simulink library "lib_Clutchless_HSC_ETE"  (R2017b)
settings: Solver=VariableStepAuto  StartTime=0.0  StopTime=10.0  RelTol=1e-3
undefined symbols (not defined in the file): cal, eng, Engine, ENGTRQ_MSMCH_Degraded_CP, ENGTRQ_MSMCH_ErrCritical_CP, ENGTRQ_MSMCH_LimpHome_CP, gb, mot, tloop
libraries: simulink x78, EC2_libraries x4, powerlib_meascontrol x2, lib_SystemDiag x1, dspsigops x1
(part 1 of 5)
settings Model: Creator=Di Russo  LastModifiedBy=Lyu19

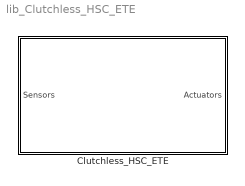
== system lib_Clutchless_HSC_ETE ==
  Clutchless_HSC_ETE : Subsystem
      mask Display: image('Images/HCU.jpg')

== system lib_Clutchless_HSC_ETE/Clutchless_HSC_ETE ==
  Sensors : Inport
  HSC : Subsystem
  Actuators : Outport
  wires:
  HSC/1(Actuators) -> Actuators/1
  Sensors/1 -> HSC/1(Sensors)

== system lib_Clutchless_HSC_ETE/Clutchless_HSC_ETE/HSC ==
  Sensors : Inport
  Camaro Fault Detection : Subsystem
  Driver_Requests : Subsystem  RequirementInfo="{'other' 'HCU_Requirements.xlsx' '@Simulink_requirement_item_5' 'true' 'Determines the  driver''s intention i.e. status of the vehicle start, HCU on/off status and the Driver Intend Axle Torque from the sensor inputs.' '' } %GIDa_ee5d0f02_0a71_4952_8ea3_2a40744828e3"
  Powertrain Manager : Subsystem
  Actuators : Outport
  wires:
  Driver_Requests/1(DriverRequests) -> Powertrain Manager/2(Driver Request)
  Camaro Fault Detection/1(Diagnostic) -> Driver_Requests/2("Diagnostic "), Powertrain Manager/3(Fault Detection)
  Powertrain Manager/1(Out1) -> Actuators/1
  Sensors/1 -> Driver_Requests/1(Sensors), Powertrain Manager/1(Sensors), Camaro Fault Detection/1(Sensors)
  Powertrain Manager/2(Controls) -> Driver_Requests/3("Controls ")

== system lib_Clutchless_HSC_ETE/Clutchless_HSC_ETE/HSC/Camaro Fault Detection ==
  Sensors : Inport
  Component Diagnostic : Subsystem
  Input Conversions : Subsystem
  Signal Diagnostic : Subsystem
  SystemDiag : lib_SystemDiag/SystemDiag
  Diagnostic : Outport
  wires:
  SystemDiag/1 -> Diagnostic/1
  Sensors/1 -> Input Conversions/1(RawSig)
  Input Conversions/1(VehSig) -> Signal Diagnostic/1(VehSig)
  Component Diagnostic/1(CompDiag) -> SystemDiag/1
  Signal Diagnostic/1(SignalDiag) -> Component Diagnostic/1(SignalDiag)

== system lib_Clutchless_HSC_ETE/Clutchless_HSC_ETE/HSC/Driver_Requests ==
  note: Driver management
  Sensors : Inport
  "Diagnostic " : Inport  Port=2
  "Controls " : Inport  Port=3
  APP_BPP to DrvIntndAxlTrq2 : Subsystem
  DriverRequests : Outport
  wires:
  Sensors/1 -> APP_BPP to DrvIntndAxlTrq2/1(Sensors)
  APP_BPP to DrvIntndAxlTrq2/1(IntndAxlTrq) -> DriverRequests/1
  "Diagnostic "/1 -> APP_BPP to DrvIntndAxlTrq2/2(Diag)
  "Controls "/1 -> APP_BPP to DrvIntndAxlTrq2/3(Controls)

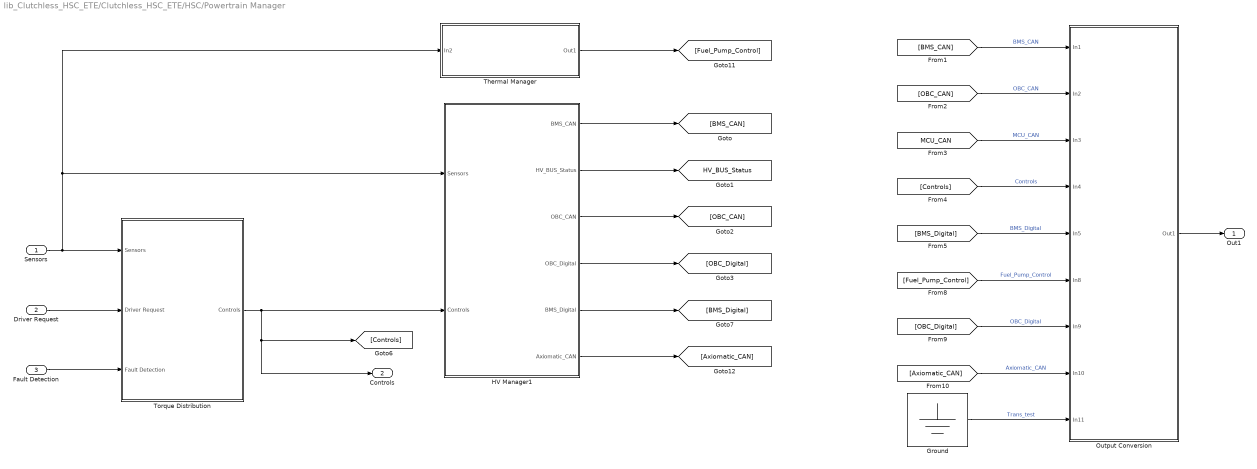
== system lib_Clutchless_HSC_ETE/Clutchless_HSC_ETE/HSC/Powertrain Manager ==
  Sensors : Inport
  Driver Request : Inport  Port=2
  Fault Detection : Inport  Port=3
  Ground : Ground
  HV Manager1 : Subsystem  AncestorBlock=lib_HVManager_PostIMG_2017a/HV Manager
  Output Conversion : Subsystem
  Thermal Manager : Subsystem  AncestorBlock=lib_ThermalManager/Thermal Manager
  Torque Distribution : Subsystem  AncestorBlock=lib_TorqueDistribution_2017a/Torque Distribution
  Out1 : Outport
  Controls : Outport  Port=2
  tag scope: HV_BUS_Status=global
  wires:
  Sensors/1 -> Torque Distribution/1(Sensors), HV Manager1/1(Sensors), Thermal Manager/1(In2)
  [Fuel_Pump_Control] -> Output Conversion/6(In8)  "Fuel_Pump_Control"
  [OBC_Digital] -> Output Conversion/7(In9)  "OBC_Digital"
  [Axiomatic_CAN] -> Output Conversion/8(In10)  "Axiomatic_CAN"
  HV Manager1/6(Axiomatic_CAN) -> [Axiomatic_CAN]
  Thermal Manager/1(Out1) -> [Fuel_Pump_Control]
  Fault Detection/1 -> Torque Distribution/3(Fault Detection)
  [BMS_Digital] -> Output Conversion/5(In5)  "BMS_Digital"
  HV Manager1/5(BMS_Digital) -> [BMS_Digital]
  Output Conversion/1(Out1) -> Out1/1
  [Controls] -> Output Conversion/4(In4)  "Controls"
  [MCU_CAN] -> Output Conversion/3(In3)  "MCU_CAN"
  [OBC_CAN] -> Output Conversion/2(In2)  "OBC_CAN"
  [BMS_CAN] -> Output Conversion/1(In1)  "BMS_CAN"
  Driver Request/1 -> Torque Distribution/2(Driver Request)
  HV Manager1/3(OBC_CAN) -> [OBC_CAN]
  HV Manager1/4(OBC_Digital) -> [OBC_Digital]
  HV Manager1/2(HV_BUS_Status) -> [HV_BUS_Status]
  HV Manager1/1(BMS_CAN) -> [BMS_CAN]
  Ground/1 -> Output Conversion/9(In11)  "Trans_test"
  Torque Distribution/1(Controls) -> HV Manager1/2(Controls), Controls/1, [Controls]

== system lib_Clutchless_HSC_ETE/Clutchless_HSC_ETE/HSC/Camaro Fault Detection/Component Diagnostic ==
  note: Component Diagnostics
  note: Component Status Setting Rule
      | xxx_CompStatus could be 0, 1, 2 or 3
      | 0: component needs to be offline
      | 1: component needs torque plant to deliver creep torque
      | 2: component needs torque plant to limit maximum torque delivery
      | 3: component needs torque plant to operate normally
  SignalDiag : Inport
  Bus Creator : BusCreator  Inputs=6
  Driver Input Diagnostic : Subsystem
  ESS Component Diagnostic : Subsystem
  Engine Component Diagnostic : Subsystem
  Override Driver Status : Subsystem
  Override ESS Status : Subsystem
  Override Engine Status : Subsystem
  Override TCM Status : Subsystem
  Transmission Component Diagnostic : Subsystem
  CompDiag : Outport
  wires:
  Engine Component Diagnostic/2(Out2) -> Bus Creator/4  "EngTrqMismchType"
  Override Driver Status/1(Out1) -> Bus Creator/1  "Driver_Input_Status"
  Override TCM Status/1(Out1) -> Bus Creator/5  "TCM_Status"
  Override Engine Status/1(Out1) -> Bus Creator/3  "ECM_Status"
  Override ESS Status/1(Out1) -> Bus Creator/2  "BMS_Status"
  Transmission Component Diagnostic/1(Out1) -> Override TCM Status/1(In1)  "TCM_CompDiag"
  Engine Component Diagnostic/1(Out1) -> Override Engine Status/1(In1)  "ECM_CompDiag"
  ESS Component Diagnostic/1(Out1) -> Override ESS Status/1(In1)  "ESS_CompDiag"
  Driver Input Diagnostic/1(Out1) -> Override Driver Status/1(In1)  "Diver_CompDiag"
  Bus Creator/1 -> CompDiag/1
  SignalDiag/1 -> Driver Input Diagnostic/1(In1), ESS Component Diagnostic/1(In1), Bus Creator/6, Transmission Component Diagnostic/1(In1), Engine Component Diagnostic/1(In1)  "RawSig"

== system lib_Clutchless_HSC_ETE/Clutchless_HSC_ETE/HSC/Camaro Fault Detection/Input Conversions ==
  note: These subsystems convert variable types to match those used in the
      | supervisor. In addition, override switches installed on each signal can
      | be used to manually override and signal for testing purposes
  note: Input Conversions and Override Switches
  RawSig : Inport
  BMS_Conversions : Subsystem
  Bus Creator : BusCreator  Inputs=5
  DriverInput_Conversions : Subsystem
  ECM_Conversions : Subsystem
  TCM_Conversions : Subsystem
  VehSig : Outport
  wires:
  TCM_Conversions/1(Out1) -> Bus Creator/4
  ECM_Conversions/1(Out1) -> Bus Creator/3
  RawSig/1 -> BMS_Conversions/1(In1), ECM_Conversions/1(In1), TCM_Conversions/1(In1), Bus Creator/5, DriverInput_Conversions/1(In1)  "RawSig"
  BMS_Conversions/1(Out1) -> Bus Creator/2
  Bus Creator/1 -> VehSig/1  "InputConvAndOvrd"
  DriverInput_Conversions/1(Out1) -> Bus Creator/1

== system lib_Clutchless_HSC_ETE/Clutchless_HSC_ETE/HSC/Camaro Fault Detection/Signal Diagnostic ==
  note: Signal Diagnostics
  note: These subsystems evaluate each signal for proper value range and other checks
  VehSig : Inport
  Bus Creator : BusCreator  Inputs=5
  Driver Signal Diagnostic : Subsystem
  ESS Signal Diagnostic : Subsystem
  Engine Signal Diagnostic : Subsystem
  Subsystem1 : Subsystem
      mask Display: fprintf('Signal Naming Rule')
  Transmission Signal Diagnostic : Subsystem
  SignalDiag : Outport
  wires:
  Bus Creator/1 -> SignalDiag/1  "SignalDiag"
  Transmission Signal Diagnostic/1(Out2) -> Bus Creator/4  "Transmission_SigDiag"
  Engine Signal Diagnostic/1(Engine_SigDiag) -> Bus Creator/3  "Engine_SigDiag"
  ESS Signal Diagnostic/1(ESS_SigDiag) -> Bus Creator/2  "ESS_SigDiag"
  Driver Signal Diagnostic/1(Driver_SigDiag) -> Bus Creator/1  "Driver_SigDiag"
  VehSig/1 -> Transmission Signal Diagnostic/1(Sensors1), Bus Creator/5, Engine Signal Diagnostic/1(Sensors1), Driver Signal Diagnostic/1(Sensors1), ESS Signal Diagnostic/1(Sensors1)

== system lib_Clutchless_HSC_ETE/Clutchless_HSC_ETE/HSC/Driver_Requests/APP_BPP to DrvIntndAxlTrq2 ==
  note: Note:Driver requested Axle Torque Calculation
  note: $Author: fy6949 $
      | $Rev: 577 $
      | $Date: 2017-1-19 08:53:15 -0500  $
  Sensors : Inport
  Diag : Inport  Port=2
  Controls : Inport  Port=3
  Bus Selector : BusSelector  OutputSignals=from_Analog.Driver_APP1,from_CAN.fromVEH_CAN.from_BCM.BrkPdlPos,from_CAN.fromEBCAN.from_ECM.VehSpdAvgDrvn,from_CAN.fromVEH_CAN.from_TCM.TrnGrRat,from_CAN.fromHV_CAN.from_MCU.INV_VCU_01.INV_Speed
  Bus Selector1 : BusSelector  OutputSignals=CompSig.RawSig.Driver_SigDiag.Drv_APP_Agree
  Bus Selector2 : BusSelector  OutputSignals=mode
  Post Driver Intnded Axle Torque : Subsystem
  Terminator : Terminator
  Terminator1 : Terminator
  IntndAxlTrq : Outport
  wires:
  Sensors/1 -> Bus Selector/1
  Controls/1 -> Bus Selector2/1
  Post Driver Intnded Axle Torque/1(IntndAxlTrq) -> IntndAxlTrq/1
  Bus Selector/2 -> Post Driver Intnded Axle Torque/2(BPP)  "<BrkPdlPos>"
  Bus Selector/3 -> Post Driver Intnded Axle Torque/3(VehicleSpeed)  "<VehSpdAvgDrvn>"
  Bus Selector/5 -> Post Driver Intnded Axle Torque/6(Motor_Speed)  "<INV_Speed>"
  Bus Selector/4 -> Post Driver Intnded Axle Torque/4(TransGearRatio)  "<TrnGrRat>"
  Bus Selector/1 -> Post Driver Intnded Axle Torque/1(APP)  "<Driver_APP1>"
  Post Driver Intnded Axle Torque/2(BrkIntndAxlTrq) -> Terminator/1
  Diag/1 -> Bus Selector1/1
  Bus Selector1/1 -> Terminator1/1  "<Drv_APP_Agree>"
  Bus Selector2/1 -> Post Driver Intnded Axle Torque/5(Mode)  "<mode>"

== system lib_Clutchless_HSC_ETE/Clutchless_HSC_ETE/HSC/Powertrain Manager/HV Manager1 ==
  Sensors : Inport
  Controls : Inport  Port=2
  Axiomatic_Output_Manager : Subsystem
  BMS_Manager : Subsystem
  Bus Creator1 : BusCreator  Inputs=4
  DCDC Manager : Subsystem
  Inverter Manager : Subsystem
  OBC_Manager : Subsystem
  BMS_CAN : Outport
  HV_BUS_Status : Outport  Port=2
  OBC_CAN : Outport  Port=3
  OBC_Digital : Outport  Port=4
  BMS_Digital : Outport  Port=5
  Axiomatic_CAN : Outport  Port=6
  tag scope: MCU_CAN=global
  wires:
  Bus Creator1/1 -> [MCU_CAN]
  Inverter Manager/2(MCU_CAN) -> Bus Creator1/2  "MCU_CAN"
  Inverter Manager/1(MCU_Status) -> [MCU_Status], Bus Creator1/1  "MCU_Status"
  Sensors/1 -> BMS_Manager/1(Sensors), DCDC Manager/1(BMSInput), Axiomatic_Output_Manager/1(Sensors), OBC_Manager/2(Sensors), Inverter Manager/2(Sensors)
  [HV_BUS_Status] -> Inverter Manager/1(HV_Bus_Status)  "HV_BUS_Status"
  [HV_BUS_Status] -> Axiomatic_Output_Manager/2(HV_Bus_Status)
  BMS_Manager/2(HV_BUS_Status) -> [HV_BUS_Status], HV_BUS_Status/1  "HV_BUS_Status"
  [HV_BUS_Status] -> OBC_Manager/1(HV_Status)
  OBC_Manager/1(OBC CAN) -> OBC_CAN/1
  OBC_Manager/2(OBC_Digital) -> OBC_Digital/1
  Controls/1 -> BMS_Manager/2(Controls), DCDC Manager/2(In1), DCDC Manager/3(In2), Inverter Manager/3(Control)
  BMS_Manager/1(BMS CAN) -> BMS_CAN/1
  BMS_Manager/3(BMS Digital) -> BMS_Digital/1
  Axiomatic_Output_Manager/1(Axiomatic_CAN) -> Axiomatic_CAN/1
  Inverter Manager/3(MCU_Relay) -> Bus Creator1/3  "MCU_Relay"
  DCDC Manager/1(Out1) -> Bus Creator1/4
  [MCU_Status] -> BMS_Manager/3(In1)

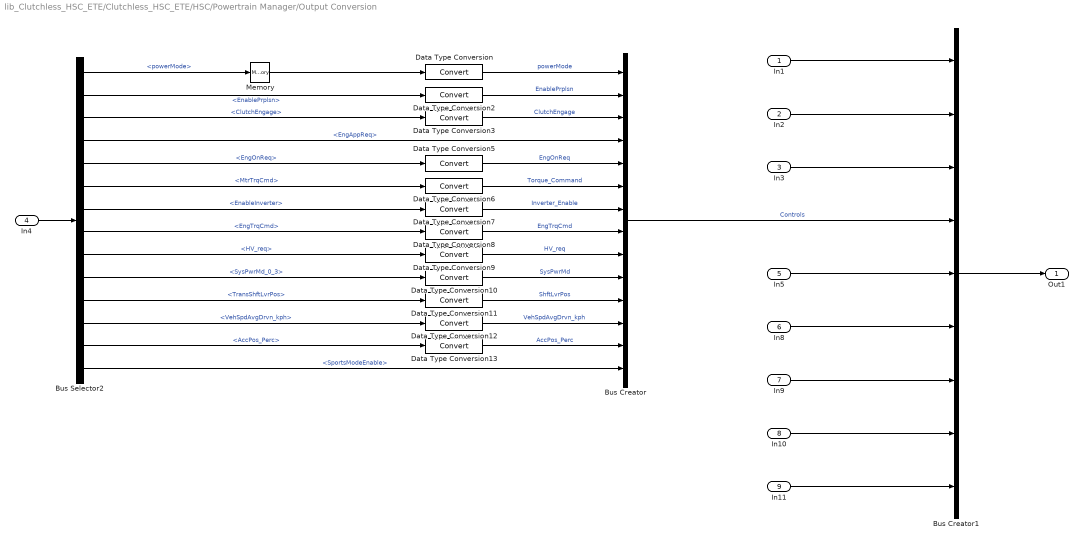
== system lib_Clutchless_HSC_ETE/Clutchless_HSC_ETE/HSC/Powertrain Manager/Output Conversion ==
  In1 : Inport
  In2 : Inport  Port=2
  In3 : Inport  Port=3
  In4 : Inport  Port=4
  In5 : Inport  Port=5
  In8 : Inport  Port=6
  In9 : Inport  Port=7
  In10 : Inport  Port=8
  In11 : Inport  Port=9
  Bus Creator : BusCreator  Inputs=14
  Bus Creator1 : BusCreator  Inputs=9
  Bus Selector2 : BusSelector  OutputSignals=powerMode,EnablePrplsn,ClutchEngage,EngAppReq,EngOnReq,MtrTrqCmd,EnableInverter,EngTrqCmd,HV_req,SysPwrMd_0_3,TransShftLvrPos,VehSpdAvgDrvn_kph,AccPos_Perc,SportsModeEnable
  Data Type Conversion{,2..3,5..13} (12 alike) : DataTypeConversion
  Memory : Memory
  Out1 : Outport
  wires:
  In10/1 -> Bus Creator1/8
  In9/1 -> Bus Creator1/7
  In8/1 -> Bus Creator1/6
  Memory/1 -> Data Type Conversion/1
  Data Type Conversion13/1 -> Bus Creator/13  "AccPos_Perc"
  Bus Selector2/13 -> Data Type Conversion13/1  "<AccPos_Perc>"
  Data Type Conversion12/1 -> Bus Creator/12  "VehSpdAvgDrvn_kph"
  Bus Selector2/12 -> Data Type Conversion12/1  "<VehSpdAvgDrvn_kph>"
  Data Type Conversion11/1 -> Bus Creator/11  "ShftLvrPos"
  Bus Selector2/11 -> Data Type Conversion11/1  "<TransShftLvrPos>"
  In5/1 -> Bus Creator1/5
  Bus Creator/1 -> Bus Creator1/4  "Controls"
  In3/1 -> Bus Creator1/3
  In2/1 -> Bus Creator1/2
  In1/1 -> Bus Creator1/1
  Bus Creator1/1 -> Out1/1
  Data Type Conversion5/1 -> Bus Creator/5  "EngOnReq"
  Data Type Conversion/1 -> Bus Creator/1  "powerMode"
  Data Type Conversion10/1 -> Bus Creator/10  "SysPwrMd"
  Data Type Conversion9/1 -> Bus Creator/9  "HV_req"
  Data Type Conversion8/1 -> Bus Creator/8  "EngTrqCmd"
  Data Type Conversion7/1 -> Bus Creator/7  "Inverter_Enable"
  Data Type Conversion6/1 -> Bus Creator/6  "Torque_Command"
  Bus Selector2/4 -> Bus Creator/4  "<EngAppReq>"
  Data Type Conversion3/1 -> Bus Creator/3  "ClutchEngage"
  Data Type Conversion2/1 -> Bus Creator/2  "EnablePrplsn"
  Bus Selector2/10 -> Data Type Conversion10/1  "<SysPwrMd_0_3>"
  Bus Selector2/9 -> Data Type Conversion9/1  "<HV_req>"
  Bus Selector2/8 -> Data Type Conversion8/1  "<EngTrqCmd>"
  Bus Selector2/7 -> Data Type Conversion7/1  "<EnableInverter>"
  Bus Selector2/6 -> Data Type Conversion6/1  "<MtrTrqCmd>"
  Bus Selector2/5 -> Data Type Conversion5/1  "<EngOnReq>"
  Bus Selector2/3 -> Data Type Conversion3/1  "<ClutchEngage>"
  Bus Selector2/2 -> Data Type Conversion2/1  "<EnablePrplsn>"
  Bus Selector2/1 -> Memory/1  "<powerMode>"
  In4/1 -> Bus Selector2/1
  In11/1 -> Bus Creator1/9
  Bus Selector2/14 -> Bus Creator/14  "<SportsModeEnable>"

== system lib_Clutchless_HSC_ETE/Clutchless_HSC_ETE/HSC/Powertrain Manager/Thermal Manager ==
  In2 : Inport
  Bus Creator : BusCreator  Inputs=3
  Bus Creator1 : BusCreator  Inputs=4
  Bus Creator2 : BusCreator  Inputs=4
  Bus Creator3 : BusCreator  Inputs=3
  Bus Creator4 : BusCreator  Inputs=1
  Bus Selector : BusSelector  OutputSignals=from_CAN.fromEBCAN.from_ECM.EngCltTmp,from_CAN.fromHV_CAN.from_BMSHybrid.BMS_Temperatur,from_CAN.fromHV_CAN.from_MCU.INV_VCU_04.INV_InverterTemperature,from_CAN.fromHV_CAN.from_MCU.INV_VCU_04.INV_ElectricMachineTemperature,from_CAN.fromEBCAN.from_ECM.EngRunAtv,from_CAN.fromHV_CAN.from_BMSHybrid.BMS_HYB_02.BMS_IstModus,from_CAN.fromVEH_CAN.from_BCM.SysPwrMd,from_CAN.fromEBCAN.from_ECM.VehSpdAvgDrvn
  Bus Selector3 : BusSelector  OutputSignals=from_CAN.fromHV_CAN.from_BMSHybrid.BMS_HYB_02.BMS_Fehler_Pilot
  Compare To Constant1 : simulink/Logic and Bit Operations/Compare To Constant  relop=>  const=0  OutDataTypeStr=boolean
  Cooling Fan Manger : Subsystem
  Data Type Conversion : DataTypeConversion  OutDataTypeStr=double
  ESS Pump Manger : Subsystem
  MotInv Pump Manger : Subsystem
  Out1 : Outport
  wires:
  Bus Selector/8 -> Bus Creator/3  "<VehSpdAvgDrvn>"
  Bus Selector/7 -> Bus Creator3/3  "<SysPwrMd>"
  Bus Selector/6 -> Bus Creator3/2  "<BMS_IstModus>"
  Bus Selector/5 -> Bus Creator3/1  "<EngRunAtv>"
  Bus Selector/4 -> Bus Creator2/4  "<INV_ElectricMachineTemperature>"
  Bus Selector/3 -> Bus Creator2/3  "<INV_InverterTemperature>"
  Bus Selector/2 -> Bus Creator2/2  "<BMS_Temperatur>"
  Bus Selector/1 -> Bus Creator2/1  "<EngCltTmp>"
  Bus Creator1/1 -> Out1/1  "Thermal_Control"
  Cooling Fan Manger/1(Fan_control) -> Bus Creator1/1  "Fan_Control"
  Bus Creator/1 -> Cooling Fan Manger/1(Temp), ESS Pump Manger/1(ESS_temp), MotInv Pump Manger/1(MotInv_temp)
  ESS Pump Manger/1(ESS_Thermal_Control) -> Bus Creator1/2  "ESS_Pump_Control"
  MotInv Pump Manger/1(MotInvpump_control) -> Bus Creator1/3  "MotMCU_Pump_Control"
  Bus Creator2/1 -> Bus Creator/1  "Temp_Signals"
  Bus Creator3/1 -> Bus Creator/2  "Component_State"
  In2/1 -> Bus Selector3/1, Bus Selector/1
  Bus Selector3/1 -> Compare To Constant1/1  "<BMS_Fehler_Pilot>"
  Bus Creator4/1 -> Bus Creator1/4  "Pump_Commands"
  Data Type Conversion/1 -> Bus Creator4/1  "FuelPump_Disable"
  Compare To Constant1/1 -> Data Type Conversion/1

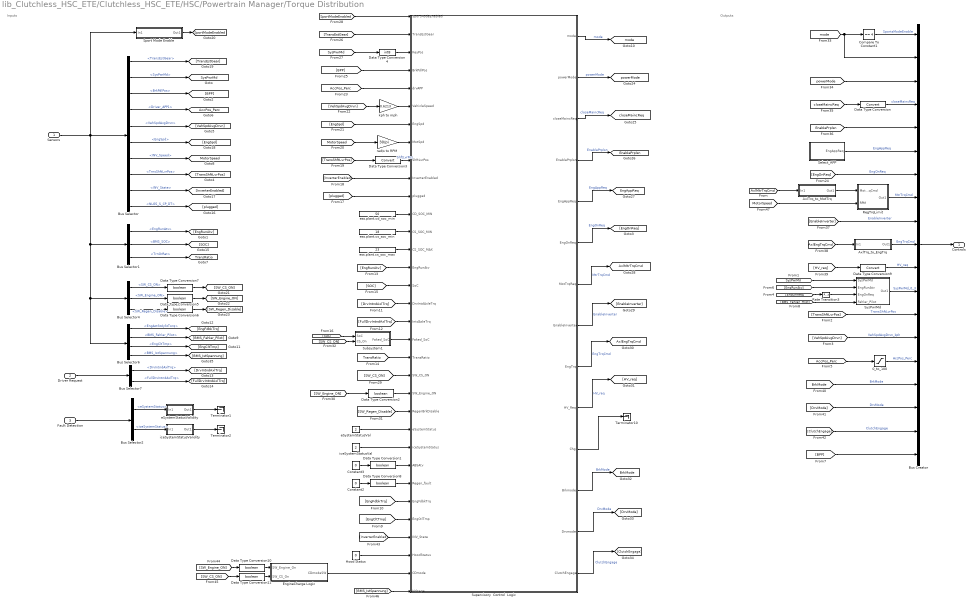
== system lib_Clutchless_HSC_ETE/Clutchless_HSC_ETE/HSC/Powertrain Manager/Torque Distribution ==
  note: Outputs
  note: Inputs
  Sensors : Inport
  Driver Request : Inport  Port=2
  Fault Detection : Inport  Port=3
  0_to_100 : Saturate  UpperLimit=100  LowerLimit=0
  AxlTrq_to_EngTrq : Subsystem
  AxlTrq_to_MotTrq : Subsystem
  Bus Creator : BusCreator  Inputs=19
  Bus Selector : BusSelector  OutputSignals=from_CAN.fromVEH_CAN.from_TCM.TransEstGear,from_CAN.fromVEH_CAN.from_BCM.SysPwrMd,from_CAN.fromVEH_CAN.from_BCM.BrkPdlPos,from_Analog.Driver_APP1,from_CAN.fromEBCAN.from_ECM.VehSpdAvgDrvn,from_CAN.fromEBCAN.from_ECM.EngSpd,from_CAN.fromHV_CAN.from_MCU.INV_VCU_01.INV_Speed,from_CAN.fromVEH_CAN.from_TCM.TrnsShftLvrPos,from_CAN.fromHV_CAN.from_MCU.INV_VCU_01.INV_State,from_CAN.fromHV_CAN.from_OBC.NLG5_ST.NLG5_S_CP_DT
  Bus Selector1 : BusSelector  OutputSignals=from_CAN.fromEBCAN.from_ECM.EngRunAtv,from_CAN.fromHV_CAN.from_BMSHybrid.BMS_SOC,from_CAN.fromVEH_CAN.from_TCM.TrnGrRat
  Bus Selector2 : BusSelector  OutputSignals=eSystemDiagOut.eSystemStatus,iceSystemDiagOut.iceSystemStatus
  Bus Selector4 : BusSelector  OutputSignals=from_Digital.SW_CS_ON,from_Digital.SW_Engine_ON,from_Digital.SW_Regen_Disable
  Bus Selector6 : BusSelector  OutputSignals=from_CAN.fromEBCAN.from_ECM.EngActStdyStTorq,from_CAN.fromHV_CAN.from_BMSHybrid.BMS_HYB_02.BMS_Fehler_Pilot,from_CAN.fromEBCAN.from_ECM.EngCltTmp,from_CAN.fromHV_CAN.from_BMSHybrid.BMS_HYB_02.BMS_IstSpannung
  Bus Selector7 : BusSelector  OutputSignals=DrvIntndAxlTrq,FullDrvIntndAxlTrq
  Compare To Constant1 : simulink/Logic and Bit Operations/Compare To Constant  relop===  const=4  OutDataTypeStr=boolean
  Constant2 : Constant  Value=0
  Constant3 : Constant  Value=0
  Data Type Conversion : DataTypeConversion
  Data Type Conversion{1..2,5..8,10..11} (8 alike) : DataTypeConversion  OutDataTypeStr=boolean
  Data Type Conversion3 : DataTypeConversion
  Data Type Conversion4 : DataTypeConversion  OutDataTypeStr=int8
  Data Type Conversion9 : DataTypeConversion
  EngineCharge Logic : Stateflow chart  TreatAsAtomicUnit=on
  Hood Status : Constant  Value=0
  Rate Transition3 : RateTransition
  RegTrqLimit : Subsystem
  Select_APP : Subsystem
  Sport Mode Enable : Subsystem
  Subsystem1 : Subsystem
  Supervisory  Control  Logic : Stateflow chart  TreatAsAtomicUnit=on
  SysPwrMd : Subsystem
  Terminator1 : Terminator
  Terminator10 : Terminator
  Terminator2 : Terminator
  eSystemStatusVal : Constant  Value=2
  eSystemStatusValidity : Subsystem
  ess.plant.cd_soc_min : Constant  Value=50
  ess.plant.cs_soc_max : Constant  Value=23
  ess.plant.cs_soc_min : Constant  Value=18
  iceSystemStatusVal : Constant  Value=2
  iceSystemStatusValidity : Subsystem
  kph to mph : Gain  Gain=0.6213
  rad/s to RPM : Gain  Gain=30/pi
  Controls : Outport
  tag scope: AccPos_Perc=global, AxlEngTrqCmd=global, AxlMtrTrqCmd=global, BrkMode=global, EnablePrplsn=global, EngAppReq=global, MotorSpeed=global, SportModeEnabled=global, SysPwrMd=global, TransRatio=global, closeMaincReq=global, mode=global, powerMode=global
  wires:
  [InverterEnabled] -> Supervisory  Control  Logic/30(INV_State)
  Data Type Conversion2/1 -> Supervisory  Control  Logic/22(SW_Engine_ON)
  [SW_Engine_ON] -> Data Type Conversion2/1
  ess.plant.cd_soc_min/1 -> Supervisory  Control  Logic/12(CD_SOC_MIN)
  ess.plant.cs_soc_min/1 -> Supervisory  Control  Logic/13(CS_SOC_MIN)
  ess.plant.cs_soc_max/1 -> Supervisory  Control  Logic/14(CS_SOC_MAX)
  Supervisory  Control  Logic/8(EnableInverter) -> [EnableInverter]  "EnableInverter"
  Supervisory  Control  Logic/4(EnablePrplsn) -> [EnablePrplsn]  "EnablePrplsn"
  Supervisory  Control  Logic/3(closeMaincReq) -> [closeMaincReq]  "closeMaincReq"
  Supervisory  Control  Logic/2(powerMode) -> [powerMode]  "powerMode"
  Supervisory  Control  Logic/1(mode) -> [mode]  "mode"
  Data Type Conversion3/1 -> Supervisory  Control  Logic/9(ShftLvrPos)  "ShftLvrPos"
  kph to mph/1 -> Supervisory  Control  Logic/6(VehicleSpeed)
  Constant2/1 -> Data Type Conversion8/1
  Supervisory  Control  Logic/11(Chg) -> Terminator10/1
  [DrvIntndAxlTrq] -> Supervisory  Control  Logic/17(DrvIntdAxleTrq)
  [FullDrvIntndAxlTrq] -> Supervisory  Control  Logic/18(IntdAxleTrq)
  Constant3/1 -> Data Type Conversion1/1
  Data Type Conversion1/1 -> Supervisory  Control  Logic/26(ABSAtv)
  Subsystem1/1(Faked_SoC) -> Supervisory  Control  Logic/19(Faked_SoC)
  Supervisory  Control  Logic/12(Brkmode) -> [BrkMode]  "BrkMode"
  Data Type Conversion8/1 -> Supervisory  Control  Logic/27(Regen_fault)
  iceSystemStatusVal/1 -> Supervisory  Control  Logic/25(iceSystemStatus)
  eSystemStatusVal/1 -> Supervisory  Control  Logic/24(eSystemStatus)
  Supervisory  Control  Logic/5(EngAppReq) -> [EngAppReq]  "EngAppReq"
  rad/s to RPM/1 -> Supervisory  Control  Logic/8(MotSpd)
  [EngCltTmp] -> Supervisory  Control  Logic/29(EngCtlTmp)
  [EngFdbkTrq] -> Supervisory  Control  Logic/28(EngFdbkTrq)
  [EngRunAtv] -> Supervisory  Control  Logic/15(EngRunAtv)
  [TransRatio] -> Supervisory  Control  Logic/20(TransRatio)
  [SOC] -> Supervisory  Control  Logic/16(SoC)
  [SOC] -> Subsystem1/1(SoC)
  [InverterEnabled] -> Supervisory  Control  Logic/10(InverterEnabled)
  [TransShftLvrPos] -> Data Type Conversion3/1
  [MotorSpeed] -> rad/s to RPM/1
  [EngSpd] -> Supervisory  Control  Logic/7(EngSpd)
  [VehSpdAvgDrvn] -> kph to mph/1
  [AccPos_Perc] -> Supervisory  Control  Logic/5(drvAPP)
  [BPP] -> Supervisory  Control  Logic/4(BrkPdlPos)
  [TransEstGear] -> Supervisory  Control  Logic/2(TransEstGear)
  [SysPwrMd] -> Data Type Conversion4/1
  Data Type Conversion4/1 -> Supervisory  Control  Logic/3(KeyPos)
  [SportModeEnabled] -> Supervisory  Control  Logic/1(SportModeEnabled)
  [SW_CS_ON] -> Supervisory  Control  Logic/21(SW_CS_ON)
  [SW_Regen_Disable] -> Supervisory  Control  Logic/23(RegenBrkDisable)
  [SW_CS_ON] -> Subsystem1/2(CS_On)
  Supervisory  Control  Logic/6(EngOnReq) -> [EngOnReq]  "EngOnReq"
  Supervisory  Control  Logic/7(MotTrqReq) -> [AxlMtrTrqCmd]  "MtrTrqCmd"
  Supervisory  Control  Logic/9(EngTrq) -> [AxlEngTrqCmd]  "EngTrqCmd"
  Supervisory  Control  Logic/10(HV_Req) -> [HV_req]  "HV_req"
  Supervisory  Control  Logic/13(Drvmode) -> [DrvMode]  "DrvMode"
  Supervisory  Control  Logic/14(ClutchEngage) -> [ClutchEngage]  "ClutchEngage"
  Bus Selector7/1 -> [DrvIntndAxlTrq]  "<DrvIntndAxlTrq>"
  Driver Request/1 -> Bus Selector7/1
  Data Type Conversion7/1 -> [SW_CS_ON]
  Bus Selector1/2 -> [SOC]  "<BMS_SOC>"
  Sport Mode Enable/1(Out1) -> [SportModeEnabled]
  Bus Selector7/2 -> [FullDrvIntndAxlTrq]  "<FullDrvIntndAxlTrq>"
  Bus Selector6/3 -> [EngCltTmp]  "<EngCltTmp>"
  Bus Selector6/2 -> [BMS_Fehler_Pilot]  "<BMS_Fehler_Pilot>"
  Bus Selector6/1 -> [EngFdbkTrq]  "<EngActStdyStTorq>"
  Data Type Conversion6/1 -> [SW_Regen_Disable]
  Data Type Conversion5/1 -> [SW_Engine_ON]
  Bus Selector/10 -> [plugged]  "<NLG5_S_CP_DT>"
  iceSystemStatusValidity/1(Out1) -> Terminator2/1
  eSystemStatusValidity/1(Out1) -> Terminator1/1
  Bus Selector4/2 -> Data Type Conversion5/1  "<SW_Engine_ON>"
  Bus Selector4/1 -> Data Type Conversion7/1  "<SW_CS_ON>"
  Bus Selector4/3 -> Data Type Conversion6/1  "<SW_Regen_Disable>"
  Bus Selector2/2 -> iceSystemStatusValidity/1(In1)  "<iceSystemStatus>"
  Bus Selector2/1 -> eSystemStatusValidity/1(In1)  "<eSystemStatus>"
  Fault Detection/1 -> Bus Selector2/1
  Bus Selector1/3 -> [TransRatio]  "<TrnGrRat>"
  Bus Selector/8 -> [TransShftLvrPos]  "<TrnsShftLvrPos>"
  Bus Selector1/1 -> [EngRunAtv]  "<EngRunAtv>"
  Bus Selector/9 -> [InverterEnabled]  "<INV_State>"
  Bus Selector/7 -> [MotorSpeed]  "<INV_Speed>"
  Bus Selector/6 -> [EngSpd]  "<EngSpd>"
  Bus Selector/5 -> [VehSpdAvgDrvn]  "<VehSpdAvgDrvn>"
  Bus Selector/4 -> [AccPos_Perc]  "<Driver_APP1>"
  Bus Selector/3 -> [BPP]  "<BrkPdlPos>"
  Bus Selector/2 -> [SysPwrMd]  "<SysPwrMd>"
  Bus Selector/1 -> [TransEstGear]  "<TransEstGear>"
  Sensors/1 -> Sport Mode Enable/1(In1), Bus Selector6/1, Bus Selector4/1, Bus Selector1/1, Bus Selector/1
  Bus Creator/1 -> Controls/1
  Rate Transition3/1 -> SysPwrMd/3(EngOnReq)
  [EngOnReq] -> Rate Transition3/1
  Data Type Conversion/1 -> Bus Creator/4  "closeMaincReq"
  [powerMode] -> Bus Creator/3
  0_to_100/1 -> Bus Creator/15  "AccPos_Perc"
  RegTrqLimit/1(Out1) -> Bus Creator/8  "MtrTrqCmd"
  [BrkMode] -> Bus Creator/16  "BrkMode"
  Select_APP/1(EngAppReq) -> Bus Creator/6  "EngAppReq"
  [HV_req] -> Data Type Conversion9/1
  [EngOnReq] -> Bus Creator/7  "EngOnReq"
  [EnableInverter] -> Bus Creator/9  "EnableInverter"
  [AccPos_Perc] -> 0_to_100/1
  [EnablePrplsn] -> Bus Creator/5
  [BMS_Fehler_Pilot] -> SysPwrMd/4(Fehler_Pilot)
  Data Type Conversion9/1 -> Bus Creator/11  "HV_req"
  [VehSpdAvgDrvn] -> Bus Creator/14  "VehSpdAvgDrvn_kph"
  SysPwrMd/1(Out1) -> Bus Creator/12  "SysPwrMd_0_3"
  [SysPwrMd] -> SysPwrMd/1(SysPwrMd)
  [DrvMode] -> Bus Creator/17  "DrvMode"
  [TransShftLvrPos] -> Bus Creator/13  "TransShftLvrPos"
  [mode] -> Bus Creator/2, Compare To Constant1/1
  [AxlEngTrqCmd] -> AxlTrq_to_EngTrq/1(In1)
  [BPP] -> Bus Creator/19
  [ClutchEngage] -> Bus Creator/18  "ClutchEngage"
  [EngRunAtv] -> SysPwrMd/2(EngRunAtv)
  Compare To Constant1/1 -> Bus Creator/1  "SportsModeEnable"
  [closeMaincReq] -> Data Type Conversion/1
  AxlTrq_to_EngTrq/1(Out1) -> Bus Creator/10  "EngTrqCmd"
  [plugged] -> Supervisory  Control  Logic/11(plugged)
  Hood Status/1 -> Supervisory  Control  Logic/31(HoodStatus)
  [MotorSpeed] -> RegTrqLimit/2(RPM)
  [AxlMtrTrqCmd] -> AxlTrq_to_MotTrq/1(In1)
  AxlTrq_to_MotTrq/1(Out1) -> RegTrqLimit/1(MotTrqCmd)
  EngineCharge Logic/1(CDmodeSW) -> Supervisory  Control  Logic/32(CDmode)
  [SW_Engine_ON] -> Data Type Conversion10/1
  Data Type Conversion10/1 -> EngineCharge Logic/1(SW_Engine_On)
  Data Type Conversion11/1 -> EngineCharge Logic/2(SW_CS_On)
  [SW_CS_ON] -> Data Type Conversion11/1
  Bus Selector6/4 -> [BMS_IstSpannung]  "<BMS_IstSpannung>"
  [BMS_IstSpannung] -> Supervisory  Control  Logic/33(Voltage)

== system lib_Clutchless_HSC_ETE/Clutchless_HSC_ETE/HSC/Camaro Fault Detection/Component Diagnostic/Driver Input Diagnostic ==
  note: APP1
      | APP2
      | BPP
      | Driver Component Status
      |
      | 1
      | 1
      | 1
      | 1
      |
      | 0
      | 1
      | 1
      | 1
      |
      | 1
      | 0
      | 1
      | 1
      |
      | 0
      | 0
      | 1
      | 0
      |
      | 1
      | 1
      | 0
      | 0
      |
      | 0
      | 0
      | 0
      | 0
  note: Driver_CompStatus
      | 1 = Component Online
      | 0 = Component Offline
  In1 : Inport
  Bus Selector : BusSelector  OutputSignals=Driver_SigDiag.Drv_APP1_[%]_SigValid,Driver_SigDiag.Drv_APP2_[%]_SigValid,Driver_SigDiag.Drv_APP_Agree,Driver_SigDiag.Drv_BPP_[%]_SigValid,Driver_SigDiag.Drv_KeyPos_[0 3]_SigValid,Driver_SigDiag.Drv_PRNDL_SigValid,Driver_SigDiag.Brake_Failed
  Driver_Input_Diag : Stateflow chart  TreatAsAtomicUnit=on
  Logical Operator : Logic  Inputs=3  AllPortsSameDT=off  OutDataTypeStr=boolean
  Out1 : Outport
  wires:
  Bus Selector/7 -> Driver_Input_Diag/5(BrakeFail)  "<Brake_Failed>"
  Bus Selector/6 -> Driver_Input_Diag/4(PRNDL)  "<Drv_PRNDL_SigValid>"
  Bus Selector/5 -> Driver_Input_Diag/3(KeyPos)  "<Drv_KeyPos_[0 3]_SigValid>"
  Bus Selector/3 -> Logical Operator/3  "<Drv_APP_Agree>"
  Logical Operator/1 -> Driver_Input_Diag/1(APP_Valid)  "APP_Valid"
  Driver_Input_Diag/1(Driver_Input_Status) -> Out1/1  "Driver_Input_Status"
  Bus Selector/4 -> Driver_Input_Diag/2(Drv_BPP_SigValid)  "<Drv_BPP_[%]_SigValid>"
  Bus Selector/2 -> Logical Operator/2  "<Drv_APP2_[%]_SigValid>"
  Bus Selector/1 -> Logical Operator/1  "<Drv_APP1_[%]_SigValid>"
  In1/1 -> Bus Selector/1

== system lib_Clutchless_HSC_ETE/Clutchless_HSC_ETE/HSC/Camaro Fault Detection/Component Diagnostic/ESS Component Diagnostic ==
  note: (Need modify)
  In1 : Inport
  BMS_CompDiag1 : Stateflow chart  TreatAsAtomicUnit=on
  Bus Selector : BusSelector  OutputSignals=ESS_SigDiag.BMS_RollingAliveActive_SigValid,ESS_SigDiag.BMS_contactorsFailed_Detected,ESS_SigDiag.BMS_essTemp_[degC]_SigValid,ESS_SigDiag.essTempRange[0_4],ESS_SigDiag.BMS_essSOC_0_1_SigValid,ESS_SigDiag.essTempRange[0_4],ESS_SigDiag.essCur_A_SigValid,ESS_SigDiag.BMSgdf_SigValid,Driver_SigDiag.Drv_KeyPos_[0 3]_SigValid
  Compare To Zero : simulink/Logic and Bit Operations/Compare To Zero  relop===  OutDataTypeStr=boolean
  Data Type Conversion : DataTypeConversion
  HVessFltReset : Constant
  Logical Operator : Logic  Operator=OR  AllPortsSameDT=off  OutDataTypeStr=boolean
  Logical Operator1 : Logic  AllPortsSameDT=off  OutDataTypeStr=boolean
  Terminator : Terminator
  Terminator1 : Terminator
  Out1 : Outport
  wires:
  [contactorsFailed_Detected] -> Logical Operator1/1
  Logical Operator1/1 -> BMS_CompDiag1/6(ess_GroundFault)
  Bus Selector/8 -> Logical Operator1/2  "<BMSgdf_SigValid>"
  Logical Operator/1 -> BMS_CompDiag1/7(ClearFault)
  HVessFltReset/1 -> Logical Operator/2
  Compare To Zero/1 -> Logical Operator/1
  Bus Selector/9 -> Compare To Zero/1  "<Drv_KeyPos_[0 3]_SigValid>"
  Bus Selector/7 -> BMS_CompDiag1/5(essCur_A_SigValid)  "<essCur_A_SigValid>"
  Bus Selector/6 -> Terminator1/1  "<essTempRange[0_4]>"
  Bus Selector/5 -> BMS_CompDiag1/4(BMS_essSOC_0_1_SigValid)  "<BMS_essSOC_0_1_SigValid>"
  Data Type Conversion/1 -> BMS_CompDiag1/3(BMS_essTemp_SigValid)  "BMS_essTemp_SigValid"
  Bus Selector/3 -> Data Type Conversion/1  "<BMS_essTemp_[degC]_SigValid>"
  Bus Selector/4 -> Terminator/1  "<essTempRange[0_4]>"
  BMS_CompDiag1/1(BMS_Status) -> Out1/1  "BMS_Status"
  Bus Selector/2 -> BMS_CompDiag1/2(BMS_contactorsFailed_SigValid), [contactorsFailed_Detected]  "<BMS_contactorsFailed_Detected>"
  Bus Selector/1 -> BMS_CompDiag1/1(BMS_RollingAliveActive_SigValid)  "<BMS_RollingAliveActive_SigValid>"
  In1/1 -> Bus Selector/1

== system lib_Clutchless_HSC_ETE/Clutchless_HSC_ETE/HSC/Camaro Fault Detection/Component Diagnostic/Engine Component Diagnostic ==
  note: Notes
  note: 0: component needs to be offline
      | 1: component needs torque plant to deliver creep torque
      | 2: component needs torque plant to limit maximum torque delivery
      | 3: component needs torque plant to operate normally
  note: add the temperature, mismatch torquesignal and have different status to the component
  note: Eng_tempRange
      | 1: normal
      | 2: high range
      | 3:above max
  note: ENGTRQ_MSMCH_Degraded_CP (40Nm): ENGTRQ_Degraded fault code.
      | ENGTRQ_MSMCH_LimpHome_CP (70Nm): ENGTRQ_LimpHome
      | ENGTRQ_MSMCH_ErrCritical_CP (100Nm): ENGTRQ_ErrCritical
  note: Eng_Torq_MsmchLevel
      | 1:Normal torque
      | 2: Limit max power
      | 3: Deliver creep torque
      | 4: offline
  In1 : Inport
  Bus Selector : BusSelector  OutputSignals=Engine_SigDiag.ECMRollingAliveActive,Engine_SigDiag.engTrqCmdRecvd_SigValid,Engine_SigDiag.ECMTrqCmd_Nm,Engine_SigDiag.EngActStdyStTorq_Nm,Engine_SigDiag.EngRunAtValid,Engine_SigDiag.Engine_Speed_rpm_SigValid,Engine_SigDiag.Eng_TempValid,Engine_SigDiag.Eng_TempRange[123],Driver_SigDiag.Drv_KeyPos_[0 3]_SigValid
  Bus Selector1 : BusSelector  OutputSignals=Eng_Torque_Mismch_Critical
  Compare To Zero : simulink/Logic and Bit Operations/Compare To Zero  relop===  OutDataTypeStr=boolean
  ECM_CompDiag : Stateflow chart  TreatAsAtomicUnit=on
  Eng_FltReset : Constant
  Eng_Torq_MsmchLevel : Stateflow chart  Commented=on  TreatAsAtomicUnit=on
  Logical Operator : Logic  Operator=OR  AllPortsSameDT=off  OutDataTypeStr=boolean
  Override  engTrqCmd : Subsystem
  Terminator1 : Terminator
  TorqMismatch Detection : Subsystem
  Out1 : Outport
  Out2 : Outport  Port=2
  wires:
  Override  engTrqCmd/1(Out1) -> ECM_CompDiag/2(engTrqCmdRecvd_SigValid)
  Bus Selector1/1 -> ECM_CompDiag/3(Eng_Torq_Msmch)  "<Eng_Torque_Mismch_Critical>"
  TorqMismatch Detection/1(Eng_Torque_Mismch) -> Out2/1, Bus Selector1/1  "EngTrqMismchType"
  Bus Selector/5 -> TorqMismatch Detection/3(In3)  "<EngRunAtValid>"
  Bus Selector/4 -> TorqMismatch Detection/2(In2)  "<EngActStdyStTorq_Nm>"
  Bus Selector/3 -> TorqMismatch Detection/1(In1)  "<ECMTrqCmd_Nm>"
  Bus Selector/8 -> ECM_CompDiag/5(Eng_TempRange_123)  "<Eng_TempRange[123]>"
  Bus Selector/7 -> Terminator1/1  "<Eng_TempValid>"
  Bus Selector/9 -> Compare To Zero/1  "<Drv_KeyPos_[0 3]_SigValid>"
  Logical Operator/1 -> ECM_CompDiag/6(ClearFault)
  Eng_FltReset/1 -> Logical Operator/2
  Compare To Zero/1 -> Logical Operator/1
  ECM_CompDiag/1(ECM_Status) -> Out1/1  "ECM_Status"
  Bus Selector/6 -> ECM_CompDiag/4(Engine_Speed_rpm_SigValid)  "<Engine_Speed_rpm_SigValid>"
  Bus Selector/2 -> Override  engTrqCmd/1(In1)  "<engTrqCmdRecvd_SigValid>"
  Bus Selector/1 -> ECM_CompDiag/1(ECM_RollingAliveActive)  "<ECMRollingAliveActive>"
  In1/1 -> Bus Selector/1

== system lib_Clutchless_HSC_ETE/Clutchless_HSC_ETE/HSC/Camaro Fault Detection/Component Diagnostic/Override Driver Status ==
  note: Override Switch Subsystem
  note: This subsystem is used to override the model value of a signal to a constant value
  In1 : Inport
  Data Type Conversion3 : DataTypeConversion
  Override Value : Constant  OutDataTypeStr=double
  Override_Driver_Status : Constant  Value=0
  Switch : Switch  Criteria=u2 > Threshold
  Out1 : Outport
  wires:
  Data Type Conversion3/1 -> Switch/3
  Override Value/1 -> Switch/1
  Switch/1 -> Out1/1
  In1/1 -> Data Type Conversion3/1
  Override_Driver_Status/1 -> Switch/2

== system lib_Clutchless_HSC_ETE/Clutchless_HSC_ETE/HSC/Camaro Fault Detection/Component Diagnostic/Override ESS Status ==
  note: Override Switch Subsystem
  note: This subsystem is used to override the model value of a signal to a constant value
  In1 : Inport
  Data Type Conversion3 : DataTypeConversion
  Override Value : Constant  Value=2  OutDataTypeStr=double
  Override_ESS_Status : Constant  Value=0
  Switch : Switch  Criteria=u2 > Threshold
  Terminator : Terminator
  Out1 : Outport
  wires:
  Data Type Conversion3/1 -> Switch/3
  Override Value/1 -> Switch/1, Out1/1
  Override_ESS_Status/1 -> Switch/2
  In1/1 -> Data Type Conversion3/1
  Switch/1 -> Terminator/1

== system lib_Clutchless_HSC_ETE/Clutchless_HSC_ETE/HSC/Camaro Fault Detection/Component Diagnostic/Override Engine Status ==
  note: Override Switch Subsystem
  note: This subsystem is used to override the model value of a signal to a constant value
  In1 : Inport
  Data Type Conversion3 : DataTypeConversion
  Override Value1 : Constant  Value=2  OutDataTypeStr=double
  Override_Engine_Status : Constant  Value=0
  Switch : Switch  Criteria=u2 > Threshold
  Terminator : Terminator
  Out1 : Outport
  wires:
  Data Type Conversion3/1 -> Switch/3
  Override_Engine_Status/1 -> Switch/2
  Override Value1/1 -> Switch/1, Out1/1
  In1/1 -> Data Type Conversion3/1
  Switch/1 -> Terminator/1

== system lib_Clutchless_HSC_ETE/Clutchless_HSC_ETE/HSC/Camaro Fault Detection/Component Diagnostic/Override TCM Status ==
  note: Override Switch Subsystem
  note: This subsystem is used to override the model value of a signal to a constant value
  In1 : Inport
  Data Type Conversion3 : DataTypeConversion
  Override Value1 : Constant  Value=2  OutDataTypeStr=double
  Override_TCM_Status : Constant  Value=0
  Switch : Switch  Criteria=u2 > Threshold
  Out1 : Outport
  wires:
  Data Type Conversion3/1 -> Switch/3
  Override Value1/1 -> Switch/1
  Override_TCM_Status/1 -> Switch/2
  Switch/1 -> Out1/1
  In1/1 -> Data Type Conversion3/1

== system lib_Clutchless_HSC_ETE/Clutchless_HSC_ETE/HSC/Camaro Fault Detection/Component Diagnostic/Transmission Component Diagnostic ==
  In1 : Inport
  Bus Selector : BusSelector  OutputSignals=Transmission_SigDiag.TCMRollingAliveActive_SigValid,Transmission_SigDiag.LvrPosTrnsShft_SigValid,Transmission_SigDiag.TransEstGear_SigValid,Transmission_SigDiag.LockupCmd_SigValid,Transmission_SigDiag.VehDirFault
  TCM_CompDia : Stateflow chart  TreatAsAtomicUnit=on
  Out1 : Outport
  wires:
  Bus Selector/5 -> TCM_CompDia/5(VehDirFault)  "<VehDirFault>"
  TCM_CompDia/1(TCM_Status) -> Out1/1  "TCM_Status"
  Bus Selector/4 -> TCM_CompDia/4(LockupCmd_SigValid)  "<LockupCmd_SigValid>"
  Bus Selector/3 -> TCM_CompDia/3(TransEstGear_SigValid)  "<TransEstGear_SigValid>"
  Bus Selector/2 -> TCM_CompDia/2(LvrPosTrnsShft_SigValid)  "<LvrPosTrnsShft_SigValid>"
  Bus Selector/1 -> TCM_CompDia/1(TCMRollingAliveActive_SigValid)  "<TCMRollingAliveActive_SigValid>"
  In1/1 -> Bus Selector/1

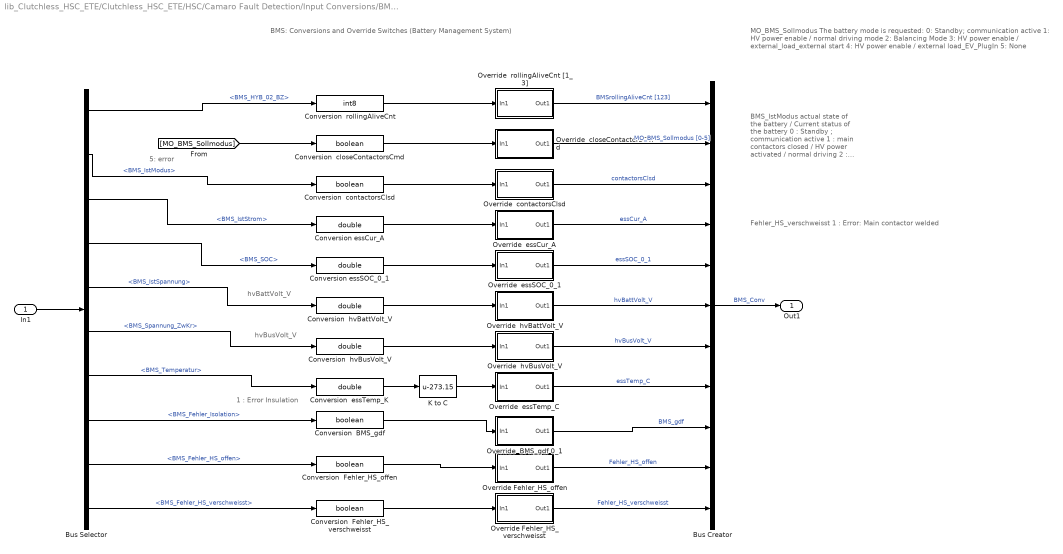
== system lib_Clutchless_HSC_ETE/Clutchless_HSC_ETE/HSC/Camaro Fault Detection/Input Conversions/BMS_Conversions ==
  note: BMS: Conversions and Override Switches
      | (Battery Management System)
  note: hvBattVolt_V
  note: hvBusVolt_V
  note: 5: error
  note: 1 : Error Insulation
  note: MO_BMS_Sollmodus
      | The battery mode is requested:
      | 0: Standby; communication active
      | 1: HV power enable / normal driving mode
      | 2: Balancing Mode
      | 3: HV power enable / external_load_external start
      | 4: HV power enable / external load_EV_PlugIn
      | 5: None
  note: BMS_IstModus
      | actual state of the battery / Current status of the battery
      | 0 : Standby ; communication active
      | 1 : main contactors closed / HV power activated / normal driving
      | 2 : closed / Balancing mode main contactors activated
      | 3 : external charging via charger High
      | 4 : external charging HV
      | 5 : Error Battery
      | 6 : External DC Charging HV
      | 7 : Init
  note: Fehler_HS_verschweisst
      | 1 : Error: Main contactor welded
  In1 : Inport
  Bus Creator : BusCreator  Inputs=11
  Bus Selector : BusSelector  OutputSignals=from_CAN.fromHV_CAN.from_BMSHybrid.BMS_HYB_02.BMS_HYB_02_BZ,from_CAN.fromHV_CAN.from_BMSHybrid.BMS_HYB_02.BMS_IstModus,from_CAN.fromHV_CAN.from_BMSHybrid.BMS_HYB_02.BMS_IstStrom,from_CAN.fromHV_CAN.from_BMSHybrid.BMS_SOC,from_CAN.fromHV_CAN.from_BMSHybrid.BMS_HYB_02.BMS_IstSpannung,from_CAN.fromHV_CAN.from_BMSHybrid.BMS_Spannung_ZwKr,from_CAN.fromHV_CAN.from_BMSHybrid.BMS_Temperatur,from_CAN.fromHV_CAN.from_BMSHybrid.BMS_Fehler_Isolation,from_CAN.fromHV_CAN.from_BMSHybrid.BMS_HYB_02.BMS_Fehler_HS_offen,from_CAN.fromHV_CAN.from_BMSHybrid.BMS_Fehler_HS_verschweisst
  Conversion  BMS_gdf : DataTypeConversion  OutDataTypeStr=boolean
  Conversion  Fehler_HS_offen : DataTypeConversion  OutDataTypeStr=boolean
  Conversion  Fehler_HS_verschweisst : DataTypeConversion  OutDataTypeStr=boolean
  Conversion  closeContactorsCmd : DataTypeConversion  OutDataTypeStr=boolean
  Conversion  contactorsClsd : DataTypeConversion  OutDataTypeStr=boolean
  Conversion  essTemp_K : DataTypeConversion  OutDataTypeStr=double
  Conversion  hvBattVolt_V : DataTypeConversion  OutDataTypeStr=double
  Conversion  hvBusVolt_V : DataTypeConversion  OutDataTypeStr=double
  Conversion  rollingAliveCnt : DataTypeConversion  OutDataTypeStr=int8
  Conversion essCur_A : DataTypeConversion  OutDataTypeStr=double
  Conversion essSOC_0_1 : DataTypeConversion  OutDataTypeStr=double
  K to C : Bias  Bias=-273.15
  Override  BMS_gdf 0_1 : Subsystem
  Override  closeContactorsCmd : Subsystem
  Override  contactorsClsd : Subsystem
  Override  essCur_A : Subsystem
  Override  essSOC_0_1 : Subsystem
  Override  essTemp_C : Subsystem
  Override  hvBattVolt_V : Subsystem
  Override  hvBusVolt_V : Subsystem
  Override  rollingAliveCnt [1_3] : Subsystem
  Override Fehler_HS_offen : Subsystem
  Override Fehler_HS_verschweisst : Subsystem
  Out1 : Outport
  wires:
  Override Fehler_HS_verschweisst/1(Out1) -> Bus Creator/11  "Fehler_HS_verschweisst"
  Conversion  Fehler_HS_verschweisst/1 -> Override Fehler_HS_verschweisst/1(In1)
  Bus Selector/10 -> Conversion  Fehler_HS_verschweisst/1  "<BMS_Fehler_HS_verschweisst>"
  Override Fehler_HS_offen/1(Out1) -> Bus Creator/10  "Fehler_HS_offen"
  Conversion  Fehler_HS_offen/1 -> Override Fehler_HS_offen/1(In1)
  Bus Selector/9 -> Conversion  Fehler_HS_offen/1  "<BMS_Fehler_HS_offen>"
  [MO_BMS_Sollmodus] -> Conversion  closeContactorsCmd/1
  Bus Selector/6 -> Conversion  hvBusVolt_V/1  "<BMS_Spannung_ZwKr>"
  Bus Selector/1 -> Conversion  rollingAliveCnt/1  "<BMS_HYB_02_BZ>"
  Bus Selector/3 -> Conversion essCur_A/1  "<BMS_IstStrom>"
  Bus Selector/4 -> Conversion essSOC_0_1/1  "<BMS_SOC>"
  Bus Selector/5 -> Conversion  hvBattVolt_V/1  "<BMS_IstSpannung>"
  Bus Selector/8 -> Conversion  BMS_gdf/1  "<BMS_Fehler_Isolation>"
  Bus Selector/7 -> Conversion  essTemp_K/1  "<BMS_Temperatur>"
  Bus Selector/2 -> Conversion  contactorsClsd/1  "<BMS_IstModus>"
  Override  BMS_gdf 0_1/1(Out1) -> Bus Creator/9  "BMS_gdf"
  Conversion  BMS_gdf/1 -> Override  BMS_gdf 0_1/1(In1)
  K to C/1 -> Override  essTemp_C/1(In1)
  Override  essTemp_C/1(Out1) -> Bus Creator/8  "essTemp_C"
  Conversion  essTemp_K/1 -> K to C/1
  Override  hvBusVolt_V/1(Out1) -> Bus Creator/7  "hvBusVolt_V"
  Override  essCur_A/1(Out1) -> Bus Creator/4  "essCur_A"
  Override  hvBattVolt_V/1(Out1) -> Bus Creator/6  "hvBattVolt_V"
  Override  essSOC_0_1/1(Out1) -> Bus Creator/5  "essSOC_0_1"
  Override  contactorsClsd/1(Out1) -> Bus Creator/3  "contactorsClsd"
  Conversion  hvBusVolt_V/1 -> Override  hvBusVolt_V/1(In1)
  Conversion  hvBattVolt_V/1 -> Override  hvBattVolt_V/1(In1)
  Conversion essSOC_0_1/1 -> Override  essSOC_0_1/1(In1)
  Conversion essCur_A/1 -> Override  essCur_A/1(In1)
  Conversion  contactorsClsd/1 -> Override  contactorsClsd/1(In1)
  Override  closeContactorsCmd/1(Out1) -> Bus Creator/2  "MO_BMS_Sollmodus [0-5]"
  Conversion  closeContactorsCmd/1 -> Override  closeContactorsCmd/1(In1)
  Bus Creator/1 -> Out1/1  "BMS_Conv"
  Override  rollingAliveCnt [1_3]/1(Out1) -> Bus Creator/1  "BMSrollingAliveCnt [123]"
  Conversion  rollingAliveCnt/1 -> Override  rollingAliveCnt [1_3]/1(In1)
  In1/1 -> Bus Selector/1

== system lib_Clutchless_HSC_ETE/Clutchless_HSC_ETE/HSC/Camaro Fault Detection/Input Conversions/DriverInput_Conversions ==
  note: Driver Controls: Conversions and Override Switches
  note: SysPwrMd (EC3)
      | 0 - Off
      | 1 -  Accessory
      | 2 - Run
      | 3 - Crank Request
  In1 : Inport
  Bus Creator : BusCreator  Inputs=7
  Bus Selector : BusSelector  OutputSignals=from_Analog.Driver_APP1,from_Analog.Driver_APP2,from_CAN.fromVEH_CAN.from_BCM.BrkPdlPos,from_CAN.fromVEH_CAN.from_BCM.SysPwrMd,from_CAN.fromVEH_CAN.from_TCM.TrnsShftLvrPos,from_CAN.fromEBCAN.from_ECM.VehSpdAvgDrvn,from_Digital.SW_Regen_Disable
  Conversion  APP1 (%) : DataTypeConversion  OutDataTypeStr=double
  Conversion  APP2 (%) : DataTypeConversion  OutDataTypeStr=double
  Conversion  BPP (%) : DataTypeConversion  OutDataTypeStr=double
  Conversion  KeyPos [0_3] : DataTypeConversion  OutDataTypeStr=int8
  Conversion  V [mph] : DataTypeConversion  OutDataTypeStr=double
  Conversion PRNDL : DataTypeConversion  OutDataTypeStr=uint8
  Conversion Regen : DataTypeConversion  OutDataTypeStr=uint8
  Override  KeyPos [0_3] : Subsystem
  Override APP (%) : Subsystem
  Override APP (%)1 : Subsystem
  Override BPP (%) : Subsystem
  Override PRNDL : Subsystem
  Override Regen : Subsystem
  Override V [mph] : Subsystem
  Out1 : Outport
  wires:
  Override Regen/1(Out1) -> Bus Creator/7  "SW_Regen"
  Conversion Regen/1 -> Override Regen/1(In1)
  Bus Selector/7 -> Conversion Regen/1  "<SW_Regen_Disable>"
  Override V [mph]/1(Out1) -> Bus Creator/6  "V [mph]"
  Conversion  V [mph]/1 -> Override V [mph]/1(In1)
  Bus Selector/6 -> Conversion  V [mph]/1  "<VehSpdAvgDrvn>"
  Conversion  APP2 (%)/1 -> Override APP (%)1/1(In1)
  Override APP (%)1/1(Out1) -> Bus Creator/2  "APP2[%]"
  Bus Selector/5 -> Conversion PRNDL/1  "<TrnsShftLvrPos>"
  Bus Selector/2 -> Conversion  APP2 (%)/1  "<Driver_APP2>"
  Override PRNDL/1(Out1) -> Bus Creator/5  "PRNDL"
  Conversion PRNDL/1 -> Override PRNDL/1(In1)
  Conversion  BPP (%)/1 -> Override BPP (%)/1(In1)
  Bus Creator/1 -> Out1/1  "DriverControls_Conv"
  Override  KeyPos [0_3]/1(Out1) -> Bus Creator/4  "keyPos [0_3]"
  Override BPP (%)/1(Out1) -> Bus Creator/3  "BPP [%]"
  Conversion  KeyPos [0_3]/1 -> Override  KeyPos [0_3]/1(In1)
  Bus Selector/4 -> Conversion  KeyPos [0_3]/1  "<SysPwrMd>"
  Bus Selector/3 -> Conversion  BPP (%)/1  "<BrkPdlPos>"
  Bus Selector/1 -> Conversion  APP1 (%)/1  "<Driver_APP1>"
  Override APP (%)/1(Out1) -> Bus Creator/1  "APP1 [%]"
  Conversion  APP1 (%)/1 -> Override APP (%)/1(In1)
  In1/1 -> Bus Selector/1

== system lib_Clutchless_HSC_ETE/Clutchless_HSC_ETE/HSC/Camaro Fault Detection/Input Conversions/ECM_Conversions ==
  note: ECM: Input Conversions and Override Switches
      | (Engine and ECM)
  In1 : Inport
  Bus Creator : BusCreator  Inputs=6
  Bus Selector : BusSelector  OutputSignals=from_CAN.fromEBCAN.from_ECM.PlatEngSpdCmdStARC,from_CAN.fromEBCAN.from_ECM.EngSpd,from_CAN.fromEBCAN.from_ECM.EngCltTmp,from_CAN.fromEBCAN.from_ECM.EngRunAtv,from_CAN.fromEBCAN.from_ECM.EngActStdyStTorq
  Conversion  ECMTrqCmd_Nm : DataTypeConversion  OutDataTypeStr=double
  Conversion  EngActStdyStTorq_Nm : DataTypeConversion  OutDataTypeStr=double
  Conversion  EngRunAtv : DataTypeConversion  OutDataTypeStr=boolean
  Conversion  Engine_Speed_rpm : DataTypeConversion  OutDataTypeStr=double
  Conversion  Engine_Temp[DegC] : DataTypeConversion  OutDataTypeStr=double
  Conversion  rollingAliveCnt : DataTypeConversion  OutDataTypeStr=int8
  Memory : Memory
  Override  ECMTrqCmd_Nm : Subsystem
  Override  ECMrollingAliveCnt : Subsystem
  Override  EngActStdyStTorq_Nm : Subsystem
  Override  EngRunAtv : Subsystem
  Override  EngineSpeed_rpm : Subsystem
  Override  Engine_Temp[DegC] : Subsystem
  Out1 : Outport
  wires:
  Memory/1 -> Conversion  ECMTrqCmd_Nm/1
  [AxlEngTrqCmd] -> Memory/1
  Bus Selector/1 -> Conversion  rollingAliveCnt/1  "<PlatEngSpdCmdStARC>"
  Override  EngActStdyStTorq_Nm/1(Out1) -> Bus Creator/6  "EngActStdyStTorq_Nm"
  Override  EngRunAtv/1(Out1) -> Bus Creator/5  "EngRunAtv"
  Override  Engine_Temp[DegC]/1(Out1) -> Bus Creator/4  "Engine_Temp[DegC]"
  Conversion  EngActStdyStTorq_Nm/1 -> Override  EngActStdyStTorq_Nm/1(In1)
  Conversion  EngRunAtv/1 -> Override  EngRunAtv/1(In1)
  Conversion  Engine_Temp[DegC]/1 -> Override  Engine_Temp[DegC]/1(In1)
  Bus Selector/5 -> Conversion  EngActStdyStTorq_Nm/1  "<EngActStdyStTorq>"
  Bus Selector/4 -> Conversion  EngRunAtv/1  "<EngRunAtv>"
  Bus Selector/3 -> Conversion  Engine_Temp[DegC]/1  "<EngCltTmp>"
  Override  EngineSpeed_rpm/1(Out1) -> Bus Creator/3  "EngineSpeed_rpm"
  Conversion  Engine_Speed_rpm/1 -> Override  EngineSpeed_rpm/1(In1)
  Bus Selector/2 -> Conversion  Engine_Speed_rpm/1  "<EngSpd>"
  Conversion  ECMTrqCmd_Nm/1 -> Override  ECMTrqCmd_Nm/1(In1)
  Override  ECMTrqCmd_Nm/1(Out1) -> Bus Creator/2  "ECMTrqCmd_Nm"
  Bus Creator/1 -> Out1/1  "ECM_Conv"
  Override  ECMrollingAliveCnt/1(Out1) -> Bus Creator/1  "ECMrollingAliveCnt [123]"
  Conversion  rollingAliveCnt/1 -> Override  ECMrollingAliveCnt/1(In1)
  In1/1 -> Bus Selector/1

== system lib_Clutchless_HSC_ETE/Clutchless_HSC_ETE/HSC/Camaro Fault Detection/Input Conversions/TCM_Conversions ==
  note: TCM: Input Conversions and Override Switches
      | (Transmission Control Module)
  In1 : Inport
  Bus Creator : BusCreator  Inputs=4
  Bus Selector : BusSelector  OutputSignals=from_CAN.fromVEH_CAN.from_TCM.TrnsShftLvrPos,from_CAN.fromVEH_CAN.from_TCM.TransEstGear,from_CAN.fromVEH_CAN.from_TCM.TrnsTrqCnvCltCmndMd
  Conversion  LockupCmd : DataTypeConversion  OutDataTypeStr=boolean
  Conversion  LvrPosTrnsShft : DataTypeConversion  OutDataTypeStr=int8
  Conversion  TransEstGear : DataTypeConversion  OutDataTypeStr=int8
  Conversion  rollingAliveCnt : DataTypeConversion  OutDataTypeStr=int8
  Override  LockupCmd : Subsystem
  "Override  LvrPosTrnsShft " : Subsystem
  Override  TransEstGear : Subsystem
  Override  rollingAliveCnt [123] : Subsystem
  TCM_RollinAliveCounter : Subsystem
  Out1 : Outport
  wires:
  TCM_RollinAliveCounter/1(Out1) -> Conversion  rollingAliveCnt/1
  In1/1 -> Bus Selector/1
  Conversion  rollingAliveCnt/1 -> Override  rollingAliveCnt [123]/1(In1)
  Override  rollingAliveCnt [123]/1(Out1) -> Bus Creator/1  "TCMrollingAliveCnt [123]"
  Bus Creator/1 -> Out1/1  "TCM_Conv"
  Bus Selector/1 -> Conversion  LvrPosTrnsShft/1  "<TrnsShftLvrPos>"
  "Override  LvrPosTrnsShft "/1(Out1) -> Bus Creator/2  "LvrPosTrnsShft"
  Conversion  LvrPosTrnsShft/1 -> "Override  LvrPosTrnsShft "/1(In1)
  Bus Selector/2 -> Conversion  TransEstGear/1  "<TransEstGear>"
  Conversion  TransEstGear/1 -> Override  TransEstGear/1(In1)
  Override  TransEstGear/1(Out1) -> Bus Creator/3  "TransEstGear"
  Bus Selector/3 -> Conversion  LockupCmd/1  "<TrnsTrqCnvCltCmndMd>"
  Conversion  LockupCmd/1 -> Override  LockupCmd/1(In1)
  Override  LockupCmd/1(Out1) -> Bus Creator/4  "LockupCmd_0_1"
